simulink model "mfbase"  (R2021a)
settings: Solver=FixedStepDiscrete  StartTime=0.0  StopTime=8  RelTol=1e-3
values from neighbouring files (symbols this model uses):
  Gain_Trans = sqrt(10/PsGu)    [Load_Analogique.m]
  Use_acc = 1    [Load_Analogique.m]
  Use_noise = 1    [Load_Analogique.m]
libraries: dsparch4 x5, dspsrcs4 x3, dspsigops x2, commanapbnd3 x1
settings Model: Creator=sebastienroy  LastModifiedBy=antho
settings SolverCC: AlgebraicLoopSolver=TrustRegion
settings DebuggingCC: SFMachineParentedDataDiag=warning

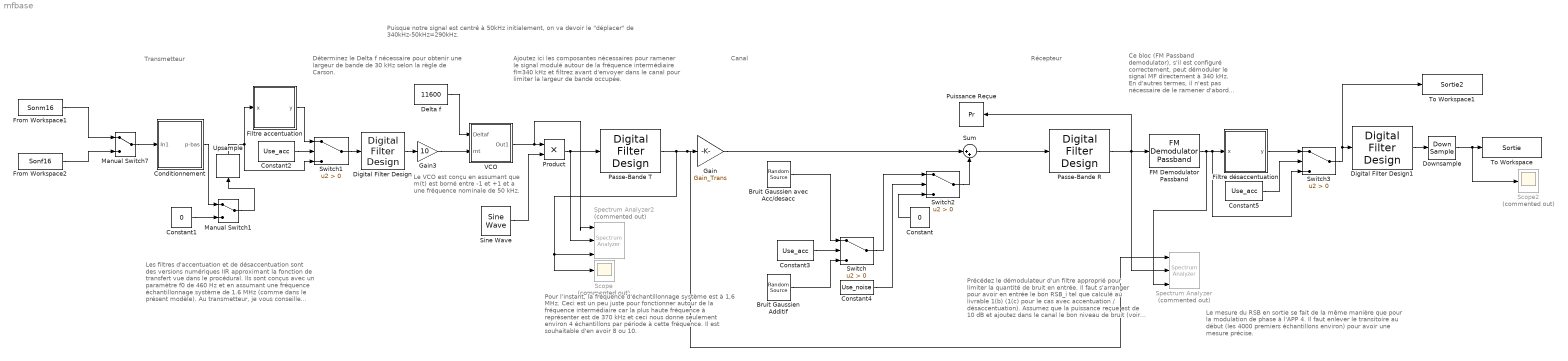
== system mfbase ==
  note: Puisque notre signal est centré à 50kHz initialement, on va devoir le "déplacer" de 340kHz-50kHz=290kHz.
  note: Les filtres d'accentuation et de désaccentuation
      | sont des versions numériques IIR approximant
      | la fonction de transfert vue dans le procédural.
      | Ils sont conçus avec un paramètre f0 de 460 Hz
      | et en assumant une fréquence échantillonnage
      | système de 1.6 MHz (comme dans le présent
      | modèle). Au transmetteur, je vous conseille d'insérer
      | le filtre d'accentuation juste après le upsample, soit
      | avant le passe-bas elliptique.
  note: Pour l'instant, la fréquence d'échantillonnage système
      | est à 1,6 MHz. Ceci est un peu juste pour fonctionner autour
      | de la fréquence intermédiaire car la plus haute fréquence
      | à représenter est de 370 kHz et ceci nous donne seulement
      | environ 4 échantillons par période à cette fréquence. Il est
      | souhaitable d'en avoir 8 ou 10.
  note: Ajoutez ici les composantes
      | nécessaires pour ramener le signal modulé autour
      | de la fréquence intermédiaire fI=340 kHz et filtrez
      | avant d'envoyer dans le canal pour limiter la largeur
      | de bande occupée.
  note: Le VCO est conçu en assumant que m(t) est borné entre -1 et +1 et a une fréquence nominale de 50 kHz.
  note: Déterminez le Delta f nécessaire pour obtenir
      | une largeur de bande de 30 kHz selon la règle
      | de Carson.
  note: Ce bloc (FM Passband demodulator), s'il est
      | configuré correctement, peut démoduler le signal
      | MF directement à 340 kHz. En d'autres termes, il
      | n'est pas nécessaire de le ramener d'abord à 50 kHz.
  note: Précédez le démodulateur d'un filtre approprié
      | pour limiter la quantité de bruit en entrée.
      |
      | Il faut s'arranger pour avoir en entrée le bon RSB_i
      | tel que calculé au livrable 1(b) (1(c) pour le cas avec
      | accentuation / désaccentuation). Assumez que la
      | puissance reçue est de 10 dB et ajoutez dans le canal
      | le bon niveau de bruit (voir livrable 1(d)).
  note: Le mesure du RSB en sortie se fait de la même manière
      | que pour la modulation de phase à l'APP 4. Il faut enlever
      | le transitoire au début (les 4000 premiers échantillons environ)
      | pour avoir une mesure précise.
  note: Transmetteur
  note: Récepteur
  note: Canal
  Bruit Gaussien Additif : dspsrcs4/Random Source  SrcType=Gaussian  NormMethod=Ziggurat  CltLength=12  MinVal=0  MaxVal=1  MeanVal=0  VarVal=1600000*(0.541251029/1000000)  RepMode=Not repeatable  rawSeed=1  IsInherit=off  SampMode=Discrete  SampTime=1/1600000  SampFrame=1  DataType=Double  OutComplex=Real  OutputFrames=off
      settings: AttributesFormatString=|
      | Variance : 1600000*(0.541251029/1000000)
      | SampleTime : %<SampTime>
      | Mean : 0
      | Method : Ziggurat
  Bruit Gaussien avec Acc/desacc : dspsrcs4/Random Source  SrcType=Gaussian  NormMethod=Ziggurat  CltLength=12  MinVal=0  MaxVal=1  MeanVal=0  VarVal=1600000*(12.23376185/1000000)  RepMode=Not repeatable  rawSeed=1  IsInherit=off  SampMode=Discrete  SampTime=1/1600000  SampFrame=1  DataType=Double  OutComplex=Real  OutputFrames=off
      settings: AttributesFormatString=|
      | Variance : 1600000*(12.23376185/1000000)
      | SampleTime : %<SampTime>
      | Mean : 0
      | Method : Ziggurat
  Conditionnement : Subsystem
  Constant : Constant  Value=0
  Constant1 : Constant  Value=0
  Constant2 : Constant  Value=Use_acc
  Constant3 : Constant  Value=Use_acc
  Constant4 : Constant  Value=Use_noise
  Constant5 : Constant  Value=Use_acc
  Delta f : Constant  Value=11600
  Digital Filter Design : dsparch4/Digital Filter Design  mwdsp_browser_bugfix_var=off
      settings: AttributesFormatString=|
      | lowpass
      | Fs: 1600kHz
      | Fpass : 3.4kHz
      | Fstop : 3.6kHz
      | IIR Elliptic
      | Apass 0.1dB
      | Astop 60dB
  Digital Filter Design1 : dsparch4/Digital Filter Design  mwdsp_browser_bugfix_var=off
      settings: AttributesFormatString=|
      | lowpass
      | Fs: 1600kHz
      | Fpass : 30kHz
      | Fstop : 33kHz
      | FIR Equiripple
      | Apass 0.1dB
      | Astop 80dB
  Downsample : DownSample  N=100  RateOptions=Allow multirate processing
  FM Demodulator Passband : commanapbnd3/FM Demodulator Passband  Fc=340000  Ph=pi/2  Kc=11600  Ho=100
      settings: SourceProductBaseCode=CM
      settings: AttributesFormatString=|
      | Carrier Freq : 340kHz
      | Phase : pi/2
      | Freq Deveation : 11600Hz
  Filtre accentuation : Subsystem
  Filtre désaccentuation : Subsystem
  From Workspace1 : FromWorkspace  VariableName=Sonm16  SampleTime=1/16000  Interpolate=off  OutputAfterFinalValue=Setting to zero
  From Workspace2 : FromWorkspace  VariableName=Sonf16  SampleTime=1/16000  Interpolate=off  OutputAfterFinalValue=Setting to zero
  Gain : Gain  Gain=Gain_Trans
      settings: AttributesFormatString=|
      | Gain
      | sqrt(10/0.126459854740914)
  Gain3 : Gain  Gain=10
  Manual Switch1 : ManualSwitch
  Manual Switch7 : ManualSwitch
  Passe-Bande R : dsparch4/Digital Filter Design  mwdsp_browser_bugfix_var=off
      settings: AttributesFormatString=|
      | Bandpass
      | Fs: 1600kHz
      | Fstop : 322kHz
      | Fpass1 : 325kHz
      | Fpass2 : 355kHz
      | Fstop2 : 358kHz
      | FIR Equiripple
      | Astop1 80dB
      | Apass 0.1dB
      | Astop2 80dB
  Passe-Bande T : dsparch4/Digital Filter Design  mwdsp_browser_bugfix_var=off
      settings: AttributesFormatString=|
      | Bandpass
      | Fs: 1600kHz
      | Fstop : 322kHz
      | Fpass1 : 325kHz
      | Fpass2 : 355kHz
      | Fstop2 : 358kHz
      | FIR Equiripple
      | Astop1 80dB
      | Apass 0.1dB
      | Astop2 80dB
  Product : Product
  Puissance Reçue : ToWorkspace  VariableName=Pr  SampleTime=-1
      settings: Save2DSignal=2-D array (concatenate along first dimension)
  Scope : Scope  Commented=on
  Scope2 : Scope  Commented=on
  Sine Wave : dspsrcs4/Sine Wave  Amplitude=1  Frequency=290000  Phase=pi/2  SampleMode=Discrete  OutComplex=Real  CompMethod=Trigonometric fcn  TableSize=Speed  SampleTime=1/1600000  SamplesPerFrame=1  ResetState=Restart at time zero  OutputFrames=off  dataType=double  wordLen=16  udDataType=sfix(16)  fracBitsMode=Best precision  numFracBits=15  OutDataTypeStr=double  LastOutDataTypeStr=double
      settings: AttributesFormatString=|
      | Amplitude %<Amplitude>
      | Fréquence %<Frequency>
      | Phase %<Phase>
      | Sample Time %<SampleTime>
  Spectrum Analyzer : SpectrumAnalyzer  Commented=on  NumInputPorts=3
  Spectrum Analyzer2 : SpectrumAnalyzer  Commented=on  NumInputPorts=3
  Sum : Sum  Inputs=|++
  Switch{,1..3} (4 alike) : Switch  Criteria=u2 > Threshold
  To Workspace : ToWorkspace  VariableName=Sortie  SampleTime=-1
      settings: Save2DSignal=2-D array (concatenate along first dimension)
  To Workspace1 : ToWorkspace  VariableName=Sortie2  SampleTime=-1
      settings: Save2DSignal=2-D array (concatenate along first dimension)
  Upsample : dspsigops/Upsample  N=10  phase=0  RateOptions=Allow multirate processing  ic=0  mode=Unused parameter value
  VCO : Subsystem
  wires:
  Manual Switch7/1 -> Conditionnement/1(In1)
  Constant1/1 -> Manual Switch1/2
  From Workspace2/1 -> Manual Switch7/2
  Conditionnement/1(p-bas) -> Manual Switch1/1
  Downsample/1 -> Scope2/1, To Workspace/1
  Manual Switch1/1 -> Upsample/1
  From Workspace1/1 -> Manual Switch7/1
  Delta f/1 -> VCO/1("Deltaf ")
  Digital Filter Design/1 -> Gain3/1
  Sine Wave/1 -> Product/2
  Product/1 -> Spectrum Analyzer2/2, Passe-Bande T/1
  Passe-Bande T/1 -> Spectrum Analyzer/1, Gain/1, Spectrum Analyzer2/3, Scope/1
  Gain3/1 -> VCO/2(mt)
  VCO/1(Out1) -> Spectrum Analyzer2/1, Product/1
  Bruit Gaussien Additif/1 -> Switch/3
  Bruit Gaussien avec Acc/desacc/1 -> Switch/1
  Switch/1 -> Switch2/1
  Constant/1 -> Switch2/3
  Switch2/1 -> Sum/2
  Sum/1 -> Passe-Bande R/1
  Constant3/1 -> Switch/2
  Upsample/1 -> Switch1/3, Filtre accentuation/1(x)
  Switch1/1 -> Digital Filter Design/1
  Filtre accentuation/1(y) -> Switch1/1
  Constant2/1 -> Switch1/2
  Constant4/1 -> Switch2/2
  FM Demodulator Passband/1 -> Spectrum Analyzer/3, Switch3/3, Filtre désaccentuation/1(x)
  Passe-Bande R/1 -> Puissance Reçue/1, Spectrum Analyzer/2, FM Demodulator Passband/1
  Constant5/1 -> Switch3/2
  Filtre désaccentuation/1(y) -> Switch3/1
  Switch3/1 -> To Workspace1/1, Digital Filter Design1/1
  Digital Filter Design1/1 -> Downsample/1
  Gain/1 -> Sum/1

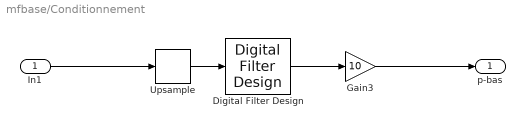
== system mfbase/Conditionnement ==
  In1 : Inport
  Digital Filter Design : dsparch4/Digital Filter Design  mwdsp_browser_bugfix_var=off
  Gain3 : Gain  Gain=10
  Upsample : dspsigops/Upsample  N=10  phase=0  RateOptions=Allow multirate processing  ic=0  mode=Unused parameter value
  p-bas : Outport
  wires:
  Upsample/1 -> Digital Filter Design/1
  Digital Filter Design/1 -> Gain3/1
  In1/1 -> Upsample/1
  Gain3/1 -> p-bas/1

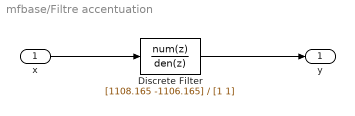
== system mfbase/Filtre accentuation ==
  x : Inport
  Discrete Filter : DiscreteFilter  Numerator=[1108.165 -1106.165]  Denominator=[1 1]
  y : Outport
  wires:
  x/1 -> Discrete Filter/1
  Discrete Filter/1 -> y/1

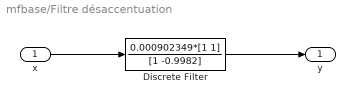
== system mfbase/Filtre désaccentuation ==
  x : Inport
  Discrete Filter : DiscreteFilter  Numerator=0.000902349*[1 1]  Denominator=[1 -0.9982]
  y : Outport
  wires:
  x/1 -> Discrete Filter/1
  Discrete Filter/1 -> y/1

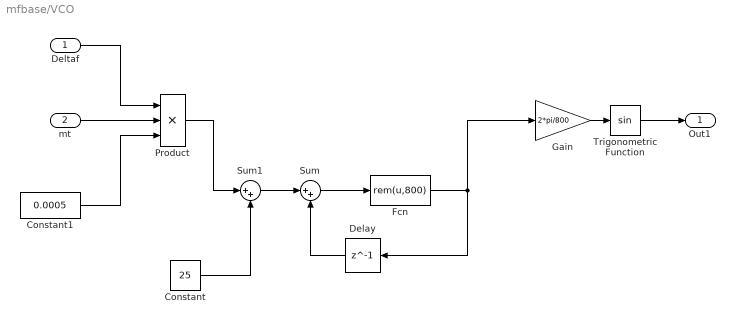
== system mfbase/VCO ==
  "Deltaf " : Inport
  mt : Inport  Port=2
  Constant : Constant  Value=25
  Constant1 : Constant  Value=0.0005
  Delay : Delay  DelayLength=1  InitialCondition=0
  Fcn : Fcn  Expr=rem(u,800)
  Gain : Gain  Gain=2*pi/800
  Product : Product  Inputs=3
  Sum : Sum  Inputs=|++
  Sum1 : Sum  Inputs=|++
  Trigonometric Function : Trigonometry
  Out1 : Outport
  wires:
  Delay/1 -> Sum/2
  Sum/1 -> Fcn/1
  Fcn/1 -> Gain/1, Delay/1
  Gain/1 -> Trigonometric Function/1
  Trigonometric Function/1 -> Out1/1
  "Deltaf "/1 -> Product/1
  mt/1 -> Product/2
  Constant1/1 -> Product/3
  Sum1/1 -> Sum/1
  Constant/1 -> Sum1/2
  Product/1 -> Sum1/1
